simulink library "xsenslib"  (R2022a)
settings: Solver=VariableStepAuto  StartTime=0.0  StopTime=10.0  RelTol=1e-3
libraries: canmsglib x48, simulink x1
(part 1 of 2)
settings Model: Creator=rodri  LastModifiedBy=rodri

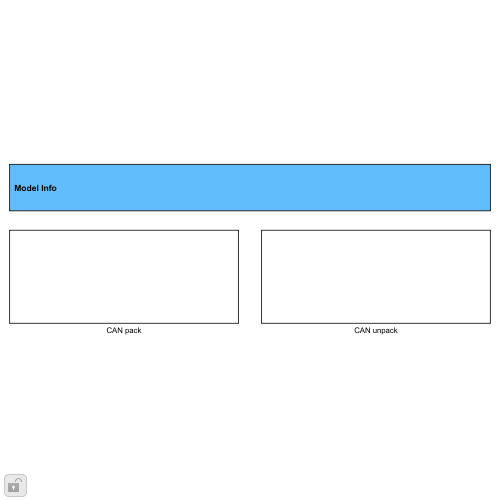
[thumbnail: Simulink's stored preview of the top-level diagram]
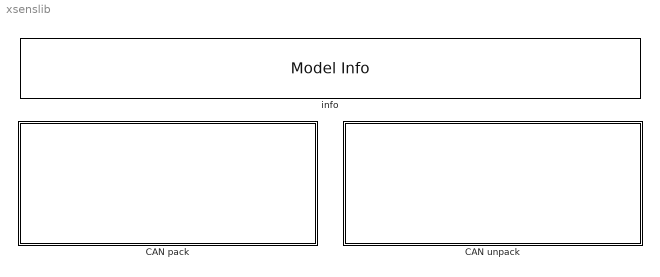
== system xsenslib ==
  CAN pack : Subsystem
  CAN unpack : Subsystem
  info : simulink/Model-Wide Utilities/Model Info  Frame=on  DisplayStringWithTags=SPEEDGOAT CAN Database Library for: xsens  HorizontalTextAlignment=Left  LeftAlignmentValue=0.01

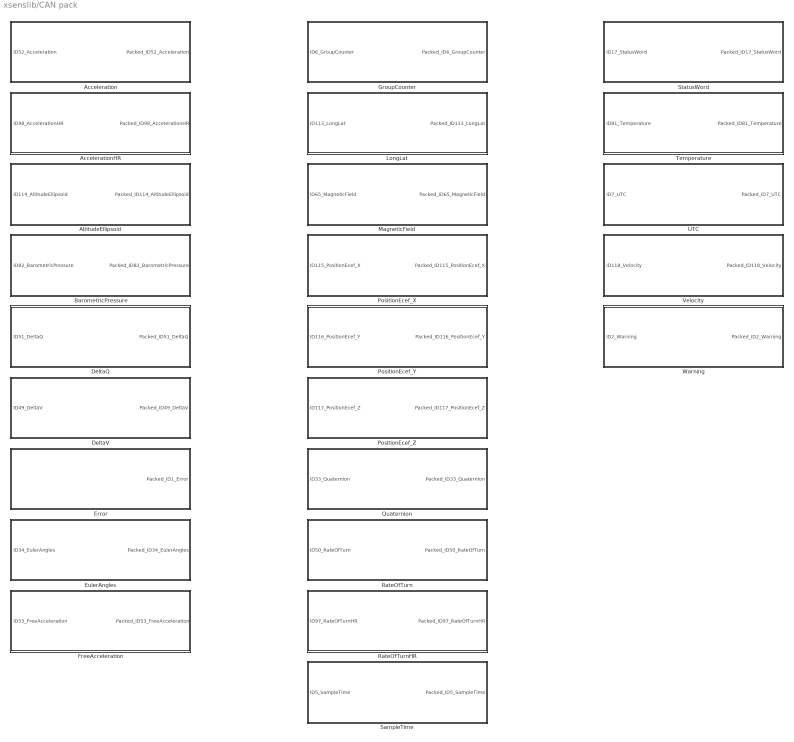
== system xsenslib/CAN pack ==
  Acceleration : Subsystem
  AccelerationHR : Subsystem
  AltitudeEllipsoid : Subsystem
  BarometricPressure : Subsystem
  DeltaQ : Subsystem
  DeltaV : Subsystem
  Error : Subsystem
  EulerAngles : Subsystem
  FreeAcceleration : Subsystem
  GroupCounter : Subsystem
  LongLat : Subsystem
  MagneticField : Subsystem
  PositionEcef_X : Subsystem
  PositionEcef_Y : Subsystem
  PositionEcef_Z : Subsystem
  Quaternion : Subsystem
  RateOfTurn : Subsystem
  RateOfTurnHR : Subsystem
  SampleTime : Subsystem
  StatusWord : Subsystem
  Temperature : Subsystem
  UTC : Subsystem
  Velocity : Subsystem
  Warning : Subsystem

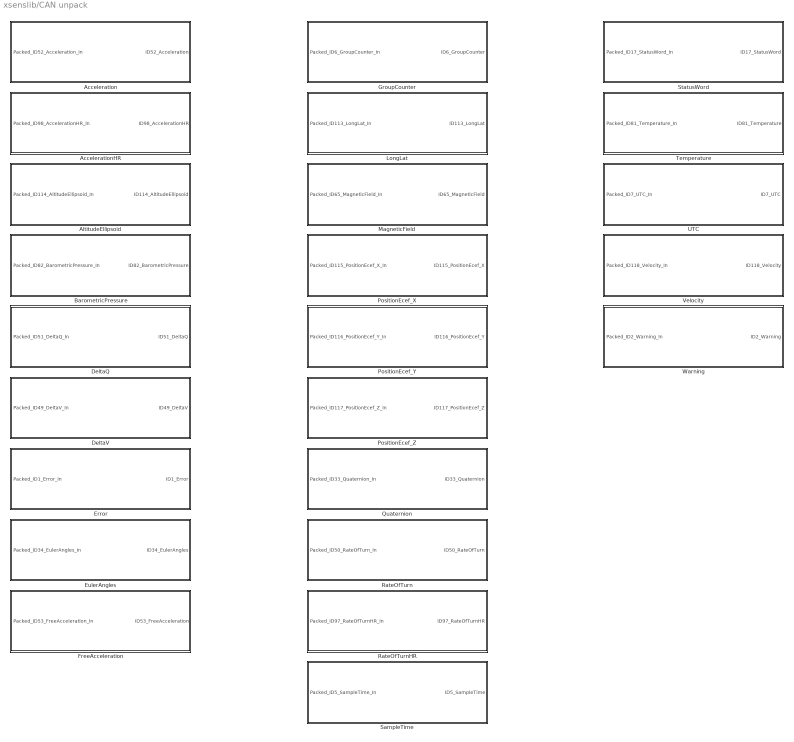
== system xsenslib/CAN unpack ==
  Acceleration : Subsystem
  AccelerationHR : Subsystem
  AltitudeEllipsoid : Subsystem
  BarometricPressure : Subsystem
  DeltaQ : Subsystem
  DeltaV : Subsystem
  Error : Subsystem
  EulerAngles : Subsystem
  FreeAcceleration : Subsystem
  GroupCounter : Subsystem
  LongLat : Subsystem
  MagneticField : Subsystem
  PositionEcef_X : Subsystem
  PositionEcef_Y : Subsystem
  PositionEcef_Z : Subsystem
  Quaternion : Subsystem
  RateOfTurn : Subsystem
  RateOfTurnHR : Subsystem
  SampleTime : Subsystem
  StatusWord : Subsystem
  Temperature : Subsystem
  UTC : Subsystem
  Velocity : Subsystem
  Warning : Subsystem

== system xsenslib/CAN pack/Acceleration ==
  In Bus Element : Inport  PortName=ID52_Acceleration  Element=accX
  In Bus Element1 : Inport  PortName=ID52_Acceleration  Element=accY
  In Bus Element2 : Inport  PortName=ID52_Acceleration  Element=accZ
  Acceleration : canmsglib/CAN Pack  CANdbFile=C:\Users\rodri\Dev\Projects\External\Tramontina\atlas\interface_models\xsens.dbc  MsgList=Acceleration  MsgName=Acceleration  MsgIDType=Standard (11-bit identifier)  MsgIdentifier=52  MsgLength=6  Remote=off  ApplyMinMax=off  BusOutput=on  SignalInfo={'accX','8','16','BE','signed','Standard','0','0.0039062','0','-100','100';'accY','24','16','BE','signed','Standard','0','0.0039062','0','-100','100';'accZ','40','16','BE','signed','Standard','0','0.0039062','0','-100','100'}
      settings: SourceProductBaseCode=XP,ME,VN  DataFormat=manually specified signals
  Packed_ID52_Acceleration : Outport
  wires:
  Acceleration/1 -> Packed_ID52_Acceleration/1
  In Bus Element/1 -> Acceleration/1
  In Bus Element1/1 -> Acceleration/2
  In Bus Element2/1 -> Acceleration/3

== system xsenslib/CAN pack/AccelerationHR ==
  In Bus Element : Inport  PortName=ID98_AccelerationHR  Element=HrAccX
  In Bus Element1 : Inport  PortName=ID98_AccelerationHR  Element=HrAccY
  In Bus Element2 : Inport  PortName=ID98_AccelerationHR  Element=HrAccZ
  AccelerationHR : canmsglib/CAN Pack  CANdbFile=C:\Users\rodri\Dev\Projects\External\Tramontina\atlas\interface_models\xsens.dbc  MsgList=AccelerationHR  MsgName=AccelerationHR  MsgIDType=Standard (11-bit identifier)  MsgIdentifier=98  MsgLength=6  Remote=off  ApplyMinMax=off  BusOutput=on  SignalInfo={'HrAccX','8','16','BE','signed','Standard','0','0.0039062','0','-100','100';'HrAccY','24','16','BE','signed','Standard','0','0.0039062','0','-100','100';'HrAccZ','40','16','BE','signed','Standard','0','0.0039062','0','-100','100'}
      settings: SourceProductBaseCode=XP,ME,VN  DataFormat=manually specified signals
  Packed_ID98_AccelerationHR : Outport
  wires:
  AccelerationHR/1 -> Packed_ID98_AccelerationHR/1
  In Bus Element/1 -> AccelerationHR/1
  In Bus Element1/1 -> AccelerationHR/2
  In Bus Element2/1 -> AccelerationHR/3

== system xsenslib/CAN pack/AltitudeEllipsoid ==
  In Bus Element : Inport  PortName=ID114_AltitudeEllipsoid  Element=altEllipsoid
  AltitudeEllipsoid : canmsglib/CAN Pack  CANdbFile=C:\Users\rodri\Dev\Projects\External\Tramontina\atlas\interface_models\xsens.dbc  MsgList=AltitudeEllipsoid  MsgName=AltitudeEllipsoid  MsgIDType=Standard (11-bit identifier)  MsgIdentifier=114  MsgLength=4  Remote=off  ApplyMinMax=off  BusOutput=on  SignalInfo={'altEllipsoid','24','32','BE','unsigned','Standard','0','3.0518e-05','0','0','50000'}
      settings: SourceProductBaseCode=XP,ME,VN  DataFormat=manually specified signals
  Packed_ID114_AltitudeEllipsoid : Outport
  wires:
  AltitudeEllipsoid/1 -> Packed_ID114_AltitudeEllipsoid/1
  In Bus Element/1 -> AltitudeEllipsoid/1

== system xsenslib/CAN pack/BarometricPressure ==
  In Bus Element : Inport  PortName=ID82_BarometricPressure  Element=Pressure
  BarometricPressure : canmsglib/CAN Pack  CANdbFile=C:\Users\rodri\Dev\Projects\External\Tramontina\atlas\interface_models\xsens.dbc  MsgList=BarometricPressure  MsgName=BarometricPressure  MsgIDType=Standard (11-bit identifier)  MsgIdentifier=82  MsgLength=4  Remote=off  ApplyMinMax=off  BusOutput=on  SignalInfo={'Pressure','24','32','BE','signed','Standard','0','3.0518e-05','0','30000','125000'}
      settings: SourceProductBaseCode=XP,ME,VN  DataFormat=manually specified signals
  Packed_ID82_BarometricPressure : Outport
  wires:
  BarometricPressure/1 -> Packed_ID82_BarometricPressure/1
  In Bus Element/1 -> BarometricPressure/1

== system xsenslib/CAN pack/DeltaQ ==
  In Bus Element : Inport  PortName=ID51_DeltaQ  Element=DeltaQ1
  In Bus Element1 : Inport  PortName=ID51_DeltaQ  Element=DeltaQ2
  In Bus Element2 : Inport  PortName=ID51_DeltaQ  Element=DeltaQ3
  In Bus Element3 : Inport  PortName=ID51_DeltaQ  Element=DeltaQ4
  DeltaQ : canmsglib/CAN Pack  CANdbFile=C:\Users\rodri\Dev\Projects\External\Tramontina\atlas\interface_models\xsens.dbc  MsgList=DeltaQ  MsgName=DeltaQ  MsgIDType=Standard (11-bit identifier)  MsgIdentifier=51  MsgLength=8  Remote=off  ApplyMinMax=off  BusOutput=on  SignalInfo={'DeltaQ1','8','16','BE','signed','Standard','0','3.0519e-05','0','-1','1';'DeltaQ2','24','16','BE','signed','Standard','0','3.0519e-05','0','-1','1';'DeltaQ3','40','16','BE','signed','Standard','0','3.0519e-05','0','-1','1';'DeltaQ4','56','16','BE','signed','Standard','0','3.0519e-05','0','-1','1'}
      settings: SourceProductBaseCode=XP,ME,VN  DataFormat=manually specified signals
  Packed_ID51_DeltaQ : Outport
  wires:
  DeltaQ/1 -> Packed_ID51_DeltaQ/1
  In Bus Element/1 -> DeltaQ/1
  In Bus Element1/1 -> DeltaQ/2
  In Bus Element2/1 -> DeltaQ/3
  In Bus Element3/1 -> DeltaQ/4

== system xsenslib/CAN pack/DeltaV ==
  In Bus Element : Inport  PortName=ID49_DeltaV  Element=Exponent
  In Bus Element1 : Inport  PortName=ID49_DeltaV  Element=X
  In Bus Element2 : Inport  PortName=ID49_DeltaV  Element=Y
  In Bus Element3 : Inport  PortName=ID49_DeltaV  Element=Z
  DeltaV : canmsglib/CAN Pack  CANdbFile=C:\Users\rodri\Dev\Projects\External\Tramontina\atlas\interface_models\xsens.dbc  MsgList=DeltaV  MsgName=DeltaV  MsgIDType=Standard (11-bit identifier)  MsgIdentifier=49  MsgLength=7  Remote=off  ApplyMinMax=off  BusOutput=on  SignalInfo={'Exponent','48','8','BE','unsigned','Standard','0','1','0','-Inf','Inf';'X','8','16','BE','signed','Standard','0','7.6294e-06','0','-0.25','0.25';'Y','24','16','BE','signed','Standard','0','7.6294e-06','0','-0.25','0.25';'Z','40','16','BE','signed','Standard','0','7.6294e-06','0','-0.25','0.25'}
      settings: SourceProductBaseCode=XP,ME,VN  DataFormat=manually specified signals
  Packed_ID49_DeltaV : Outport
  wires:
  DeltaV/1 -> Packed_ID49_DeltaV/1
  In Bus Element/1 -> DeltaV/1
  In Bus Element1/1 -> DeltaV/2
  In Bus Element2/1 -> DeltaV/3
  In Bus Element3/1 -> DeltaV/4

== system xsenslib/CAN pack/Error ==
  Error : canmsglib/CAN Pack  CANdbFile=C:\Users\rodri\Dev\Projects\External\Tramontina\atlas\interface_models\xsens.dbc  MsgList=Error  MsgName=Error  MsgIDType=Standard (11-bit identifier)  MsgIdentifier=1  MsgLength=1  Remote=off  ApplyMinMax=off  BusOutput=on  SignalInfo={}
      settings: SourceProductBaseCode=XP,ME,VN  DataFormat=manually specified signals
  Ground : Ground
  Packed_ID1_Error : Outport
  wires:
  Error/1 -> Packed_ID1_Error/1
  Ground/1 -> Error/1

== system xsenslib/CAN pack/EulerAngles ==
  In Bus Element : Inport  PortName=ID34_EulerAngles  Element=pitch
  In Bus Element1 : Inport  PortName=ID34_EulerAngles  Element=roll
  In Bus Element2 : Inport  PortName=ID34_EulerAngles  Element=yaw
  EulerAngles : canmsglib/CAN Pack  CANdbFile=C:\Users\rodri\Dev\Projects\External\Tramontina\atlas\interface_models\xsens.dbc  MsgList=EulerAngles  MsgName=EulerAngles  MsgIDType=Standard (11-bit identifier)  MsgIdentifier=34  MsgLength=6  Remote=off  ApplyMinMax=off  BusOutput=on  SignalInfo={'pitch','24','16','BE','signed','Standard','0','0.0078125','0','-90','90';'roll','8','16','BE','signed','Standard','0','0.0078125','0','-180','180';'yaw','40','16','BE','signed','Standard','0','0.0078125','0','-180','180'}
      settings: SourceProductBaseCode=XP,ME,VN  DataFormat=manually specified signals
  Packed_ID34_EulerAngles : Outport
  wires:
  EulerAngles/1 -> Packed_ID34_EulerAngles/1
  In Bus Element/1 -> EulerAngles/1
  In Bus Element1/1 -> EulerAngles/2
  In Bus Element2/1 -> EulerAngles/3

== system xsenslib/CAN pack/FreeAcceleration ==
  In Bus Element : Inport  PortName=ID53_FreeAcceleration  Element=FreeAccX
  In Bus Element1 : Inport  PortName=ID53_FreeAcceleration  Element=FreeAccY
  In Bus Element2 : Inport  PortName=ID53_FreeAcceleration  Element=FreeAccZ
  FreeAcceleration : canmsglib/CAN Pack  CANdbFile=C:\Users\rodri\Dev\Projects\External\Tramontina\atlas\interface_models\xsens.dbc  MsgList=FreeAcceleration  MsgName=FreeAcceleration  MsgIDType=Standard (11-bit identifier)  MsgIdentifier=53  MsgLength=6  Remote=off  ApplyMinMax=off  BusOutput=on  SignalInfo={'FreeAccX','8','16','BE','signed','Standard','0','0.0039062','0','-100','100';'FreeAccY','24','16','BE','signed','Standard','0','0.0039062','0','-100','100';'FreeAccZ','40','16','BE','signed','Standard','0','0.0039062','0','-100','100'}
      settings: SourceProductBaseCode=XP,ME,VN  DataFormat=manually specified signals
  Packed_ID53_FreeAcceleration : Outport
  wires:
  FreeAcceleration/1 -> Packed_ID53_FreeAcceleration/1
  In Bus Element/1 -> FreeAcceleration/1
  In Bus Element1/1 -> FreeAcceleration/2
  In Bus Element2/1 -> FreeAcceleration/3

== system xsenslib/CAN pack/GroupCounter ==
  In Bus Element : Inport  PortName=ID6_GroupCounter  Element=Counter
  GroupCounter : canmsglib/CAN Pack  CANdbFile=C:\Users\rodri\Dev\Projects\External\Tramontina\atlas\interface_models\xsens.dbc  MsgList=GroupCounter  MsgName=GroupCounter  MsgIDType=Standard (11-bit identifier)  MsgIdentifier=6  MsgLength=2  Remote=off  ApplyMinMax=off  BusOutput=on  SignalInfo={'Counter','8','16','BE','unsigned','Standard','0','1','0','-Inf','Inf'}
      settings: SourceProductBaseCode=XP,ME,VN  DataFormat=manually specified signals
  Packed_ID6_GroupCounter : Outport
  wires:
  GroupCounter/1 -> Packed_ID6_GroupCounter/1
  In Bus Element/1 -> GroupCounter/1

== system xsenslib/CAN pack/LongLat ==
  In Bus Element : Inport  PortName=ID113_LongLat  Element=latitude
  In Bus Element1 : Inport  PortName=ID113_LongLat  Element=longitude
  LongLat : canmsglib/CAN Pack  CANdbFile=C:\Users\rodri\Dev\Projects\External\Tramontina\atlas\interface_models\xsens.dbc  MsgList=LongLat  MsgName=LongLat  MsgIDType=Standard (11-bit identifier)  MsgIdentifier=113  MsgLength=8  Remote=off  ApplyMinMax=off  BusOutput=on  SignalInfo={'latitude','24','32','BE','signed','Standard','0','5.9605e-08','0','-90','90';'longitude','56','32','BE','signed','Standard','0','1.1921e-07','0','-180','180'}
      settings: SourceProductBaseCode=XP,ME,VN  DataFormat=manually specified signals
  Packed_ID113_LongLat : Outport
  wires:
  LongLat/1 -> Packed_ID113_LongLat/1
  In Bus Element/1 -> LongLat/1
  In Bus Element1/1 -> LongLat/2

== system xsenslib/CAN pack/MagneticField ==
  In Bus Element : Inport  PortName=ID65_MagneticField  Element=magX
  In Bus Element1 : Inport  PortName=ID65_MagneticField  Element=magY
  In Bus Element2 : Inport  PortName=ID65_MagneticField  Element=magZ
  MagneticField : canmsglib/CAN Pack  CANdbFile=C:\Users\rodri\Dev\Projects\External\Tramontina\atlas\interface_models\xsens.dbc  MsgList=MagneticField  MsgName=MagneticField  MsgIDType=Standard (11-bit identifier)  MsgIdentifier=65  MsgLength=6  Remote=off  ApplyMinMax=off  BusOutput=on  SignalInfo={'magX','8','16','BE','signed','Standard','0','0.00097656','0','-32','32';'magY','24','16','BE','signed','Standard','0','0.00097656','0','-32','32';'magZ','40','16','BE','signed','Standard','0','0.00097656','0','-32','32'}
      settings: SourceProductBaseCode=XP,ME,VN  DataFormat=manually specified signals
  Packed_ID65_MagneticField : Outport
  wires:
  MagneticField/1 -> Packed_ID65_MagneticField/1
  In Bus Element/1 -> MagneticField/1
  In Bus Element1/1 -> MagneticField/2
  In Bus Element2/1 -> MagneticField/3

== system xsenslib/CAN pack/PositionEcef_X ==
  In Bus Element : Inport  PortName=ID115_PositionEcef_X  Element=PositionEcef_X
  PositionEcef_X : canmsglib/CAN Pack  CANdbFile=C:\Users\rodri\Dev\Projects\External\Tramontina\atlas\interface_models\xsens.dbc  MsgList=PositionEcef_X  MsgName=PositionEcef_X  MsgIDType=Standard (11-bit identifier)  MsgIdentifier=115  MsgLength=4  Remote=off  ApplyMinMax=off  BusOutput=on  SignalInfo={'PositionEcef_X','24','32','BE','signed','Standard','0','0.0039062','0','-6500000','6500000'}
      settings: SourceProductBaseCode=XP,ME,VN  DataFormat=manually specified signals
  Packed_ID115_PositionEcef_X : Outport
  wires:
  PositionEcef_X/1 -> Packed_ID115_PositionEcef_X/1
  In Bus Element/1 -> PositionEcef_X/1

== system xsenslib/CAN pack/PositionEcef_Y ==
  In Bus Element : Inport  PortName=ID116_PositionEcef_Y  Element=PositionEcef_Y
  PositionEcef_Y : canmsglib/CAN Pack  CANdbFile=C:\Users\rodri\Dev\Projects\External\Tramontina\atlas\interface_models\xsens.dbc  MsgList=PositionEcef_Y  MsgName=PositionEcef_Y  MsgIDType=Standard (11-bit identifier)  MsgIdentifier=116  MsgLength=4  Remote=off  ApplyMinMax=off  BusOutput=on  SignalInfo={'PositionEcef_Y','24','32','BE','signed','Standard','0','0.0039062','0','-6500000','6500000'}
      settings: SourceProductBaseCode=XP,ME,VN  DataFormat=manually specified signals
  Packed_ID116_PositionEcef_Y : Outport
  wires:
  PositionEcef_Y/1 -> Packed_ID116_PositionEcef_Y/1
  In Bus Element/1 -> PositionEcef_Y/1

== system xsenslib/CAN pack/PositionEcef_Z ==
  In Bus Element : Inport  PortName=ID117_PositionEcef_Z  Element=PositionEcef_Z
  PositionEcef_Z : canmsglib/CAN Pack  CANdbFile=C:\Users\rodri\Dev\Projects\External\Tramontina\atlas\interface_models\xsens.dbc  MsgList=PositionEcef_Z  MsgName=PositionEcef_Z  MsgIDType=Standard (11-bit identifier)  MsgIdentifier=117  MsgLength=4  Remote=off  ApplyMinMax=off  BusOutput=on  SignalInfo={'PositionEcef_Z','24','32','BE','signed','Standard','0','0.0039062','0','-6500000','6500000'}
      settings: SourceProductBaseCode=XP,ME,VN  DataFormat=manually specified signals
  Packed_ID117_PositionEcef_Z : Outport
  wires:
  PositionEcef_Z/1 -> Packed_ID117_PositionEcef_Z/1
  In Bus Element/1 -> PositionEcef_Z/1

== system xsenslib/CAN pack/Quaternion ==
  In Bus Element : Inport  PortName=ID33_Quaternion  Element=Q1
  In Bus Element1 : Inport  PortName=ID33_Quaternion  Element=Q2
  In Bus Element2 : Inport  PortName=ID33_Quaternion  Element=Q3
  In Bus Element3 : Inport  PortName=ID33_Quaternion  Element=Q4
  Quaternion : canmsglib/CAN Pack  CANdbFile=C:\Users\rodri\Dev\Projects\External\Tramontina\atlas\interface_models\xsens.dbc  MsgList=Quaternion  MsgName=Quaternion  MsgIDType=Standard (11-bit identifier)  MsgIdentifier=33  MsgLength=8  Remote=off  ApplyMinMax=off  BusOutput=on  SignalInfo={'Q1','8','16','BE','signed','Standard','0','3.0518e-05','0','-1','1';'Q2','24','16','BE','signed','Standard','0','3.0518e-05','0','-1','1';'Q3','40','16','BE','signed','Standard','0','3.0518e-05','0','-1','1';'Q4','56','16','BE','signed','Standard','0','3.0518e-05','0','-Inf','Inf'}
      settings: SourceProductBaseCode=XP,ME,VN  DataFormat=manually specified signals
  Packed_ID33_Quaternion : Outport
  wires:
  Quaternion/1 -> Packed_ID33_Quaternion/1
  In Bus Element/1 -> Quaternion/1
  In Bus Element1/1 -> Quaternion/2
  In Bus Element2/1 -> Quaternion/3
  In Bus Element3/1 -> Quaternion/4

== system xsenslib/CAN pack/RateOfTurn ==
  In Bus Element : Inport  PortName=ID50_RateOfTurn  Element=gyrX
  In Bus Element1 : Inport  PortName=ID50_RateOfTurn  Element=gyrY
  In Bus Element2 : Inport  PortName=ID50_RateOfTurn  Element=gyrZ
  RateOfTurn : canmsglib/CAN Pack  CANdbFile=C:\Users\rodri\Dev\Projects\External\Tramontina\atlas\interface_models\xsens.dbc  MsgList=RateOfTurn  MsgName=RateOfTurn  MsgIDType=Standard (11-bit identifier)  MsgIdentifier=50  MsgLength=6  Remote=off  ApplyMinMax=off  BusOutput=on  SignalInfo={'gyrX','8','16','BE','signed','Standard','0','0.0019531','0','-Inf','Inf';'gyrY','24','16','BE','signed','Standard','0','0.0019531','0','-Inf','Inf';'gyrZ','40','16','BE','signed','Standard','0','0.0019531','0','-Inf','Inf'}
      settings: SourceProductBaseCode=XP,ME,VN  DataFormat=manually specified signals
  Packed_ID50_RateOfTurn : Outport
  wires:
  RateOfTurn/1 -> Packed_ID50_RateOfTurn/1
  In Bus Element/1 -> RateOfTurn/1
  In Bus Element1/1 -> RateOfTurn/2
  In Bus Element2/1 -> RateOfTurn/3

== system xsenslib/CAN pack/RateOfTurnHR ==
  In Bus Element : Inport  PortName=ID97_RateOfTurnHR  Element=HrGyrX
  In Bus Element1 : Inport  PortName=ID97_RateOfTurnHR  Element=HrGyrY
  In Bus Element2 : Inport  PortName=ID97_RateOfTurnHR  Element=HrGyrZ
  RateOfTurnHR : canmsglib/CAN Pack  CANdbFile=C:\Users\rodri\Dev\Projects\External\Tramontina\atlas\interface_models\xsens.dbc  MsgList=RateOfTurnHR  MsgName=RateOfTurnHR  MsgIDType=Standard (11-bit identifier)  MsgIdentifier=97  MsgLength=6  Remote=off  ApplyMinMax=off  BusOutput=on  SignalInfo={'HrGyrX','8','16','BE','signed','Standard','0','0.0019531','0','-Inf','Inf';'HrGyrY','24','16','BE','signed','Standard','0','0.0019531','0','-Inf','Inf';'HrGyrZ','40','16','BE','signed','Standard','0','0.0019531','0','-Inf','Inf'}
      settings: SourceProductBaseCode=XP,ME,VN  DataFormat=manually specified signals
  Packed_ID97_RateOfTurnHR : Outport
  wires:
  RateOfTurnHR/1 -> Packed_ID97_RateOfTurnHR/1
  In Bus Element/1 -> RateOfTurnHR/1
  In Bus Element1/1 -> RateOfTurnHR/2
  In Bus Element2/1 -> RateOfTurnHR/3

== system xsenslib/CAN pack/SampleTime ==
  In Bus Element : Inport  PortName=ID5_SampleTime  Element=Timestamp
  SampleTime : canmsglib/CAN Pack  CANdbFile=C:\Users\rodri\Dev\Projects\External\Tramontina\atlas\interface_models\xsens.dbc  MsgList=SampleTime  MsgName=SampleTime  MsgIDType=Standard (11-bit identifier)  MsgIdentifier=5  MsgLength=4  Remote=off  ApplyMinMax=off  BusOutput=on  SignalInfo={'Timestamp','24','32','BE','unsigned','Standard','0','1','0','-Inf','Inf'}
      settings: SourceProductBaseCode=XP,ME,VN  DataFormat=manually specified signals
  Packed_ID5_SampleTime : Outport
  wires:
  SampleTime/1 -> Packed_ID5_SampleTime/1
  In Bus Element/1 -> SampleTime/1

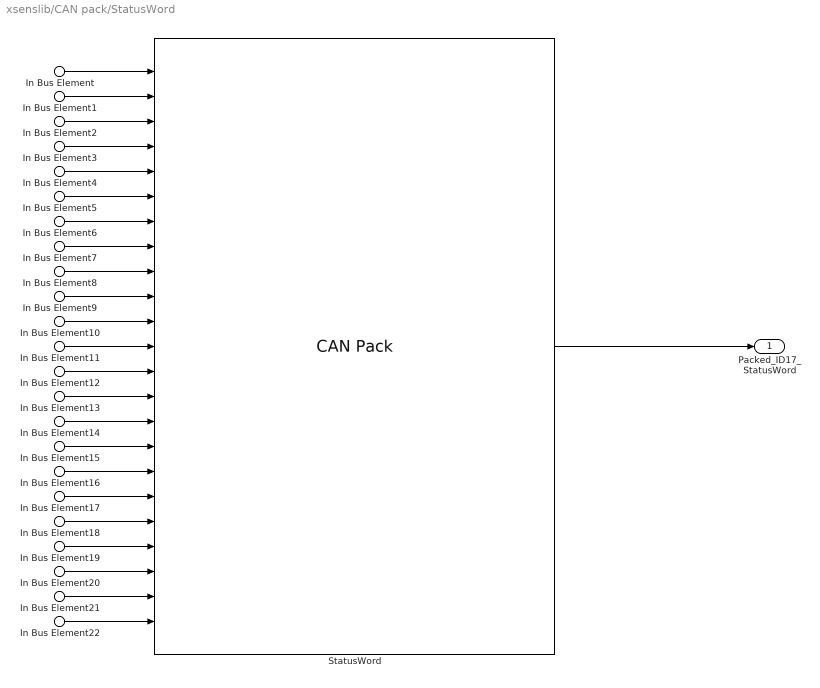
== system xsenslib/CAN pack/StatusWord ==
  In Bus Element : Inport  PortName=ID17_StatusWord  Element=ClipAccX
  In Bus Element1 : Inport  PortName=ID17_StatusWord  Element=ClipAccY
  In Bus Element2 : Inport  PortName=ID17_StatusWord  Element=ClipAccZ
  In Bus Element3 : Inport  PortName=ID17_StatusWord  Element=ClipGyrX
  In Bus Element4 : Inport  PortName=ID17_StatusWord  Element=ClipGyrY
  In Bus Element5 : Inport  PortName=ID17_StatusWord  Element=ClipGyrZ
  In Bus Element6 : Inport  PortName=ID17_StatusWord  Element=ClipMagX
  In Bus Element7 : Inport  PortName=ID17_StatusWord  Element=ClipMagY
  In Bus Element8 : Inport  PortName=ID17_StatusWord  Element=ClipMagZ
  In Bus Element9 : Inport  PortName=ID17_StatusWord  Element=ClippingDetected
  In Bus Element10 : Inport  PortName=ID17_StatusWord  Element=ExternalClockSynced
  In Bus Element11 : Inport  PortName=ID17_StatusWord  Element=FilterMode
  In Bus Element12 : Inport  PortName=ID17_StatusWord  Element=GpsValid
  In Bus Element13 : Inport  PortName=ID17_StatusWord  Element=HaveGnssTimePulse
  In Bus Element14 : Inport  PortName=ID17_StatusWord  Element=Interpolated
  In Bus Element15 : Inport  PortName=ID17_StatusWord  Element=NoRotation
  In Bus Element16 : Inport  PortName=ID17_StatusWord  Element=OrientationValid
  In Bus Element17 : Inport  PortName=ID17_StatusWord  Element=RepresentativeMotion
  In Bus Element18 : Inport  PortName=ID17_StatusWord  Element=Retransmitted
  In Bus Element19 : Inport  PortName=ID17_StatusWord  Element=RtkStatus
  In Bus Element20 : Inport  PortName=ID17_StatusWord  Element=SelfTestOk
  In Bus Element21 : Inport  PortName=ID17_StatusWord  Element=SyncIn
  In Bus Element22 : Inport  PortName=ID17_StatusWord  Element=SyncOut
  StatusWord : canmsglib/CAN Pack  CANdbFile=C:\Users\rodri\Dev\Projects\External\Tramontina\atlas\interface_models\xsens.dbc  MsgList=StatusWord  MsgName=StatusWord  MsgIDType=Standard (11-bit identifier)  MsgIdentifier=17  MsgLength=4  Remote=off  ApplyMinMax=off  BusOutput=on  SignalInfo={'ClipAccX','16','1','LE','unsigned','Standard','0','1','0','0','1';'ClipAccY','17','1','LE','unsigned','Standard','0','1','0','0','1';'ClipAccZ','18','1','LE','unsigned','Standard','0','1','0','0','1';'ClipGyrX','19','1','LE','unsigned','Standard','0','1','0','0','1';'ClipGyrY','20','1','LE','unsigned','Standard','0','1','0','0','1';'ClipGyrZ','21','1','LE','unsigned','Standard','0','1','0','0','1';'ClipMagX','22','1','LE','unsigned','Standard','0','1','0','0','1';'ClipMagY','23','1','LE','unsigned','Standard','0','1','0','0','1';'ClipMagZ','8','1','LE','unsigned','Standard','0','1','0','0','1';'ClippingDetected','11','1','LE','unsigned','Standard','0','1','0','0','1';'ExternalClockSynced','30','1','LE','unsigned','Standard','0','1','0','0','1';'FilterMode','15','3','BE','unsigned','Standard','0','1','0','0','1';'GpsValid','26','1','LE','unsigned','Standard','0','1','0','0','1';'HaveGnssTimePulse','2','1','LE','unsigned','Standard','0','1','0','0','1';'Interpolated','12','1','LE','unsigned','Standard','0','1','0','0','1';'NoRotation','27','2','BE','unsigned','Standard','0','1','0','0','3';'OrientationValid','25','1','LE','unsigned','Standard','0','1','0','0','1';'RepresentativeMotion','29','1','LE','unsigned','Standard','0','1','0','0','1';'Retransmitted','10','1','LE','unsigned','Standard','0','1','0','0','1';'RtkStatus','3','2','BE','unsigned','Standard','0','1','0','0','1';'SelfTestOk','24','1','LE','unsigned','Standard','0','1','0','0','1';'SyncIn','13','1','LE','unsigned','Standard','0','1','0','0','1';'SyncOut','14','1','LE','unsigned','Standard','0','1','0','0','1'}
      settings: SourceProductBaseCode=XP,ME,VN  DataFormat=manually specified signals
  Packed_ID17_StatusWord : Outport
  wires:
  StatusWord/1 -> Packed_ID17_StatusWord/1
  In Bus Element/1 -> StatusWord/1
  In Bus Element1/1 -> StatusWord/2
  In Bus Element2/1 -> StatusWord/3
  In Bus Element3/1 -> StatusWord/4
  In Bus Element4/1 -> StatusWord/5
  In Bus Element5/1 -> StatusWord/6
  In Bus Element6/1 -> StatusWord/7
  In Bus Element7/1 -> StatusWord/8
  In Bus Element8/1 -> StatusWord/9
  In Bus Element9/1 -> StatusWord/10
  In Bus Element10/1 -> StatusWord/11
  In Bus Element11/1 -> StatusWord/12
  In Bus Element12/1 -> StatusWord/13
  In Bus Element13/1 -> StatusWord/14
  In Bus Element14/1 -> StatusWord/15
  In Bus Element15/1 -> StatusWord/16
  In Bus Element16/1 -> StatusWord/17
  In Bus Element17/1 -> StatusWord/18
  In Bus Element18/1 -> StatusWord/19
  In Bus Element19/1 -> StatusWord/20
  In Bus Element20/1 -> StatusWord/21
  In Bus Element21/1 -> StatusWord/22
  In Bus Element22/1 -> StatusWord/23

== system xsenslib/CAN pack/Temperature ==
  In Bus Element : Inport  PortName=ID81_Temperature  Element=Temperature
  Temperature : canmsglib/CAN Pack  CANdbFile=C:\Users\rodri\Dev\Projects\External\Tramontina\atlas\interface_models\xsens.dbc  MsgList=Temperature  MsgName=Temperature  MsgIDType=Standard (11-bit identifier)  MsgIdentifier=81  MsgLength=2  Remote=off  ApplyMinMax=off  BusOutput=on  SignalInfo={'Temperature','8','16','BE','signed','Standard','0','0.0039062','0','-40','85'}
      settings: SourceProductBaseCode=XP,ME,VN  DataFormat=manually specified signals
  Packed_ID81_Temperature : Outport
  wires:
  Temperature/1 -> Packed_ID81_Temperature/1
  In Bus Element/1 -> Temperature/1

== system xsenslib/CAN pack/UTC ==
  In Bus Element : Inport  PortName=ID7_UTC  Element=day
  In Bus Element1 : Inport  PortName=ID7_UTC  Element=hour
  In Bus Element2 : Inport  PortName=ID7_UTC  Element=minute
  In Bus Element3 : Inport  PortName=ID7_UTC  Element=month
  In Bus Element4 : Inport  PortName=ID7_UTC  Element=second
  In Bus Element5 : Inport  PortName=ID7_UTC  Element=tenthms
  In Bus Element6 : Inport  PortName=ID7_UTC  Element=year
  UTC : canmsglib/CAN Pack  CANdbFile=C:\Users\rodri\Dev\Projects\External\Tramontina\atlas\interface_models\xsens.dbc  MsgList=UTC  MsgName=UTC  MsgIDType=Standard (11-bit identifier)  MsgIdentifier=7  MsgLength=8  Remote=off  ApplyMinMax=off  BusOutput=on  SignalInfo={'day','16','8','BE','unsigned','Standard','0','1','0','1','31';'hour','24','8','BE','unsigned','Standard','0','1','0','0','24';'minute','32','8','BE','unsigned','Standard','0','1','0','0','60';'month','8','8','BE','unsigned','Standard','0','1','0','1','12';'second','40','8','BE','unsigned','Standard','0','1','0','0','60';'tenthms','56','16','BE','unsigned','Standard','0','1','0','-Inf','Inf';'year','0','8','BE','unsigned','Standard','0','1','0','-Inf','Inf'}
      settings: SourceProductBaseCode=XP,ME,VN  DataFormat=manually specified signals
  Packed_ID7_UTC : Outport
  wires:
  UTC/1 -> Packed_ID7_UTC/1
  In Bus Element/1 -> UTC/1
  In Bus Element1/1 -> UTC/2
  In Bus Element2/1 -> UTC/3
  In Bus Element3/1 -> UTC/4
  In Bus Element4/1 -> UTC/5
  In Bus Element5/1 -> UTC/6
  In Bus Element6/1 -> UTC/7

== system xsenslib/CAN pack/Velocity ==
  In Bus Element : Inport  PortName=ID118_Velocity  Element=velX
  In Bus Element1 : Inport  PortName=ID118_Velocity  Element=velY
  In Bus Element2 : Inport  PortName=ID118_Velocity  Element=velZ
  Velocity : canmsglib/CAN Pack  CANdbFile=C:\Users\rodri\Dev\Projects\External\Tramontina\atlas\interface_models\xsens.dbc  MsgList=Velocity  MsgName=Velocity  MsgIDType=Standard (11-bit identifier)  MsgIdentifier=118  MsgLength=6  Remote=off  ApplyMinMax=off  BusOutput=on  SignalInfo={'velX','8','16','BE','signed','Standard','0','0.015625','0','-500','500';'velY','24','16','BE','signed','Standard','0','0.015625','0','-500','500';'velZ','40','16','BE','signed','Standard','0','0.015625','0','-500','500'}
      settings: SourceProductBaseCode=XP,ME,VN  DataFormat=manually specified signals
  Packed_ID118_Velocity : Outport
  wires:
  Velocity/1 -> Packed_ID118_Velocity/1
  In Bus Element/1 -> Velocity/1
  In Bus Element1/1 -> Velocity/2
  In Bus Element2/1 -> Velocity/3

== system xsenslib/CAN pack/Warning ==
  In Bus Element : Inport  PortName=ID2_Warning  Element=WarningCode
  Warning : canmsglib/CAN Pack  CANdbFile=C:\Users\rodri\Dev\Projects\External\Tramontina\atlas\interface_models\xsens.dbc  MsgList=Warning  MsgName=Warning  MsgIDType=Standard (11-bit identifier)  MsgIdentifier=2  MsgLength=1  Remote=off  ApplyMinMax=off  BusOutput=on  SignalInfo={'WarningCode','0','8','BE','unsigned','Standard','0','1','0','-Inf','Inf'}
      settings: SourceProductBaseCode=XP,ME,VN  DataFormat=manually specified signals
  Packed_ID2_Warning : Outport
  wires:
  Warning/1 -> Packed_ID2_Warning/1
  In Bus Element/1 -> Warning/1

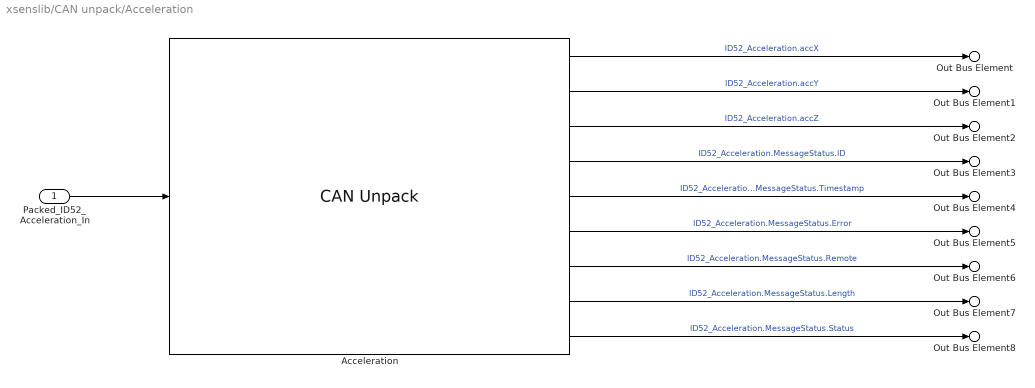
== system xsenslib/CAN unpack/Acceleration ==
  Packed_ID52_Acceleration_In : Inport
  Acceleration : canmsglib/CAN Unpack  CANdbFile=C:\Users\rodri\Dev\Projects\External\Tramontina\atlas\interface_models\xsens.dbc  MsgList=Acceleration  MsgName=Acceleration  MsgIDType=Standard (11-bit identifier)  MsgIdentifier=52  MsgLength=6  SignalInfo={'accX','8','16','BE','signed','Standard','0','0.0039062','0','-100','100';'accY','24','16','BE','signed','Standard','0','0.0039062','0','-100','100';'accZ','40','16','BE','signed','Standard','0','0.0039062','0','-100','100'}  IDPort=on  TimestampPort=on  ErrorPort=on  RemotePort=on  LengthPort=on  StatusPort=on  ApplyMinMax=off
      settings: SourceProductBaseCode=XP,ME,VN
  Out Bus Element : Outport  PortName=ID52_Acceleration  Element=accX
  Out Bus Element1 : Outport  PortName=ID52_Acceleration  Element=accY
  Out Bus Element2 : Outport  PortName=ID52_Acceleration  Element=accZ
  Out Bus Element3 : Outport  PortName=ID52_Acceleration  Element=MessageStatus.ID
  Out Bus Element4 : Outport  PortName=ID52_Acceleration  Element=MessageStatus.Timestamp
  Out Bus Element5 : Outport  PortName=ID52_Acceleration  Element=MessageStatus.Error
  Out Bus Element6 : Outport  PortName=ID52_Acceleration  Element=MessageStatus.Remote
  Out Bus Element7 : Outport  PortName=ID52_Acceleration  Element=MessageStatus.Length
  Out Bus Element8 : Outport  PortName=ID52_Acceleration  Element=MessageStatus.Status
  wires:
  Packed_ID52_Acceleration_In/1 -> Acceleration/1
  Acceleration/1 -> Out Bus Element/1  "ID52_Acceleration.accX"
  Acceleration/2 -> Out Bus Element1/1  "ID52_Acceleration.accY"
  Acceleration/3 -> Out Bus Element2/1  "ID52_Acceleration.accZ"
  Acceleration/4 -> Out Bus Element3/1  "ID52_Acceleration.MessageStatus.ID"
  Acceleration/5 -> Out Bus Element4/1  "ID52_Acceleration.MessageStatus.Timestamp"
  Acceleration/6 -> Out Bus Element5/1  "ID52_Acceleration.MessageStatus.Error"
  Acceleration/7 -> Out Bus Element6/1  "ID52_Acceleration.MessageStatus.Remote"
  Acceleration/8 -> Out Bus Element7/1  "ID52_Acceleration.MessageStatus.Length"
  Acceleration/9 -> Out Bus Element8/1  "ID52_Acceleration.MessageStatus.Status"

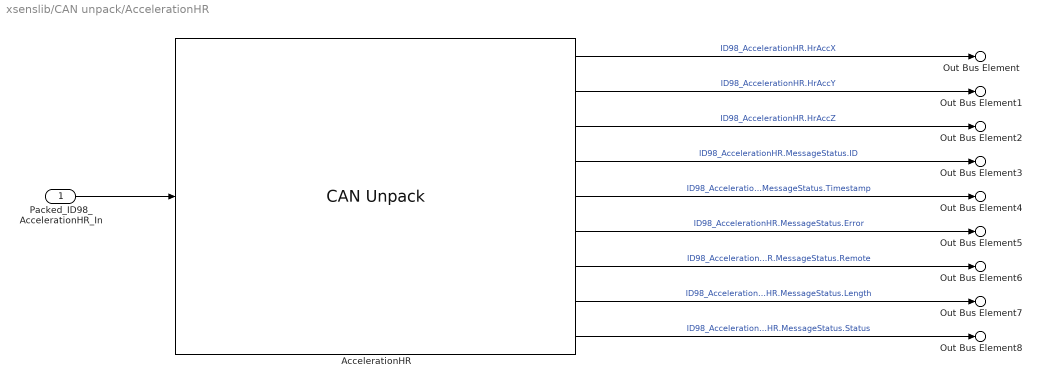
== system xsenslib/CAN unpack/AccelerationHR ==
  Packed_ID98_AccelerationHR_In : Inport
  AccelerationHR : canmsglib/CAN Unpack  CANdbFile=C:\Users\rodri\Dev\Projects\External\Tramontina\atlas\interface_models\xsens.dbc  MsgList=AccelerationHR  MsgName=AccelerationHR  MsgIDType=Standard (11-bit identifier)  MsgIdentifier=98  MsgLength=6  SignalInfo={'HrAccX','8','16','BE','signed','Standard','0','0.0039062','0','-100','100';'HrAccY','24','16','BE','signed','Standard','0','0.0039062','0','-100','100';'HrAccZ','40','16','BE','signed','Standard','0','0.0039062','0','-100','100'}  IDPort=on  TimestampPort=on  ErrorPort=on  RemotePort=on  LengthPort=on  StatusPort=on  ApplyMinMax=off
      settings: SourceProductBaseCode=XP,ME,VN
  Out Bus Element : Outport  PortName=ID98_AccelerationHR  Element=HrAccX
  Out Bus Element1 : Outport  PortName=ID98_AccelerationHR  Element=HrAccY
  Out Bus Element2 : Outport  PortName=ID98_AccelerationHR  Element=HrAccZ
  Out Bus Element3 : Outport  PortName=ID98_AccelerationHR  Element=MessageStatus.ID
  Out Bus Element4 : Outport  PortName=ID98_AccelerationHR  Element=MessageStatus.Timestamp
  Out Bus Element5 : Outport  PortName=ID98_AccelerationHR  Element=MessageStatus.Error
  Out Bus Element6 : Outport  PortName=ID98_AccelerationHR  Element=MessageStatus.Remote
  Out Bus Element7 : Outport  PortName=ID98_AccelerationHR  Element=MessageStatus.Length
  Out Bus Element8 : Outport  PortName=ID98_AccelerationHR  Element=MessageStatus.Status
  wires:
  Packed_ID98_AccelerationHR_In/1 -> AccelerationHR/1
  AccelerationHR/1 -> Out Bus Element/1  "ID98_AccelerationHR.HrAccX"
  AccelerationHR/2 -> Out Bus Element1/1  "ID98_AccelerationHR.HrAccY"
  AccelerationHR/3 -> Out Bus Element2/1  "ID98_AccelerationHR.HrAccZ"
  AccelerationHR/4 -> Out Bus Element3/1  "ID98_AccelerationHR.MessageStatus.ID"
  AccelerationHR/5 -> Out Bus Element4/1  "ID98_AccelerationHR.MessageStatus.Timestamp"
  AccelerationHR/6 -> Out Bus Element5/1  "ID98_AccelerationHR.MessageStatus.Error"
  AccelerationHR/7 -> Out Bus Element6/1  "ID98_AccelerationHR.MessageStatus.Remote"
  AccelerationHR/8 -> Out Bus Element7/1  "ID98_AccelerationHR.MessageStatus.Length"
  AccelerationHR/9 -> Out Bus Element8/1  "ID98_AccelerationHR.MessageStatus.Status"

== system xsenslib/CAN unpack/AltitudeEllipsoid ==
  Packed_ID114_AltitudeEllipsoid_In : Inport
  AltitudeEllipsoid : canmsglib/CAN Unpack  CANdbFile=C:\Users\rodri\Dev\Projects\External\Tramontina\atlas\interface_models\xsens.dbc  MsgList=AltitudeEllipsoid  MsgName=AltitudeEllipsoid  MsgIDType=Standard (11-bit identifier)  MsgIdentifier=114  MsgLength=4  SignalInfo={'altEllipsoid','24','32','BE','unsigned','Standard','0','3.0518e-05','0','0','50000'}  IDPort=on  TimestampPort=on  ErrorPort=on  RemotePort=on  LengthPort=on  StatusPort=on  ApplyMinMax=off
      settings: SourceProductBaseCode=XP,ME,VN
  Out Bus Element : Outport  PortName=ID114_AltitudeEllipsoid  Element=altEllipsoid
  Out Bus Element1 : Outport  PortName=ID114_AltitudeEllipsoid  Element=MessageStatus.ID
  Out Bus Element2 : Outport  PortName=ID114_AltitudeEllipsoid  Element=MessageStatus.Timestamp
  Out Bus Element3 : Outport  PortName=ID114_AltitudeEllipsoid  Element=MessageStatus.Error
  Out Bus Element4 : Outport  PortName=ID114_AltitudeEllipsoid  Element=MessageStatus.Remote
  Out Bus Element5 : Outport  PortName=ID114_AltitudeEllipsoid  Element=MessageStatus.Length
  Out Bus Element6 : Outport  PortName=ID114_AltitudeEllipsoid  Element=MessageStatus.Status
  wires:
  Packed_ID114_AltitudeEllipsoid_In/1 -> AltitudeEllipsoid/1
  AltitudeEllipsoid/1 -> Out Bus Element/1  "ID114_AltitudeEllipsoid.altEllipsoid"
  AltitudeEllipsoid/2 -> Out Bus Element1/1  "ID114_AltitudeEllipsoid.MessageStatus.ID"
  AltitudeEllipsoid/3 -> Out Bus Element2/1  "ID114_AltitudeEllipsoid.MessageStatus.Timestamp"
  AltitudeEllipsoid/4 -> Out Bus Element3/1  "ID114_AltitudeEllipsoid.MessageStatus.Error"
  AltitudeEllipsoid/5 -> Out Bus Element4/1  "ID114_AltitudeEllipsoid.MessageStatus.Remote"
  AltitudeEllipsoid/6 -> Out Bus Element5/1  "ID114_AltitudeEllipsoid.MessageStatus.Length"
  AltitudeEllipsoid/7 -> Out Bus Element6/1  "ID114_AltitudeEllipsoid.MessageStatus.Status"

== system xsenslib/CAN unpack/BarometricPressure ==
  Packed_ID82_BarometricPressure_In : Inport
  BarometricPressure : canmsglib/CAN Unpack  CANdbFile=C:\Users\rodri\Dev\Projects\External\Tramontina\atlas\interface_models\xsens.dbc  MsgList=BarometricPressure  MsgName=BarometricPressure  MsgIDType=Standard (11-bit identifier)  MsgIdentifier=82  MsgLength=4  SignalInfo={'Pressure','24','32','BE','signed','Standard','0','3.0518e-05','0','30000','125000'}  IDPort=on  TimestampPort=on  ErrorPort=on  RemotePort=on  LengthPort=on  StatusPort=on  ApplyMinMax=off
      settings: SourceProductBaseCode=XP,ME,VN
  Out Bus Element : Outport  PortName=ID82_BarometricPressure  Element=Pressure
  Out Bus Element1 : Outport  PortName=ID82_BarometricPressure  Element=MessageStatus.ID
  Out Bus Element2 : Outport  PortName=ID82_BarometricPressure  Element=MessageStatus.Timestamp
  Out Bus Element3 : Outport  PortName=ID82_BarometricPressure  Element=MessageStatus.Error
  Out Bus Element4 : Outport  PortName=ID82_BarometricPressure  Element=MessageStatus.Remote
  Out Bus Element5 : Outport  PortName=ID82_BarometricPressure  Element=MessageStatus.Length
  Out Bus Element6 : Outport  PortName=ID82_BarometricPressure  Element=MessageStatus.Status
  wires:
  Packed_ID82_BarometricPressure_In/1 -> BarometricPressure/1
  BarometricPressure/1 -> Out Bus Element/1  "ID82_BarometricPressure.Pressure"
  BarometricPressure/2 -> Out Bus Element1/1  "ID82_BarometricPressure.MessageStatus.ID"
  BarometricPressure/3 -> Out Bus Element2/1  "ID82_BarometricPressure.MessageStatus.Timestamp"
  BarometricPressure/4 -> Out Bus Element3/1  "ID82_BarometricPressure.MessageStatus.Error"
  BarometricPressure/5 -> Out Bus Element4/1  "ID82_BarometricPressure.MessageStatus.Remote"
  BarometricPressure/6 -> Out Bus Element5/1  "ID82_BarometricPressure.MessageStatus.Length"
  BarometricPressure/7 -> Out Bus Element6/1  "ID82_BarometricPressure.MessageStatus.Status"

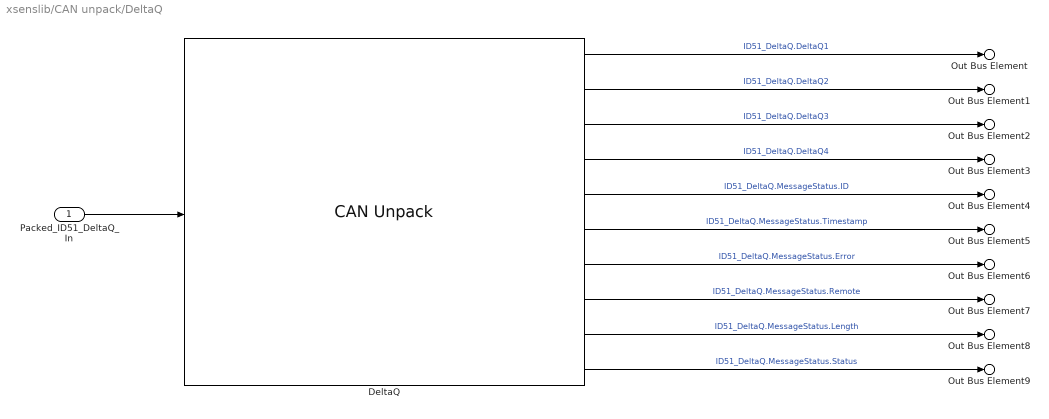
== system xsenslib/CAN unpack/DeltaQ ==
  Packed_ID51_DeltaQ_In : Inport
  DeltaQ : canmsglib/CAN Unpack  CANdbFile=C:\Users\rodri\Dev\Projects\External\Tramontina\atlas\interface_models\xsens.dbc  MsgList=DeltaQ  MsgName=DeltaQ  MsgIDType=Standard (11-bit identifier)  MsgIdentifier=51  MsgLength=8  SignalInfo={'DeltaQ1','8','16','BE','signed','Standard','0','3.0519e-05','0','-1','1';'DeltaQ2','24','16','BE','signed','Standard','0','3.0519e-05','0','-1','1';'DeltaQ3','40','16','BE','signed','Standard','0','3.0519e-05','0','-1','1';'DeltaQ4','56','16','BE','signed','Standard','0','3.0519e-05','0','-1','1'}  IDPort=on  TimestampPort=on  ErrorPort=on  RemotePort=on  LengthPort=on  StatusPort=on  ApplyMinMax=off
      settings: SourceProductBaseCode=XP,ME,VN
  Out Bus Element : Outport  PortName=ID51_DeltaQ  Element=DeltaQ1
  Out Bus Element1 : Outport  PortName=ID51_DeltaQ  Element=DeltaQ2
  Out Bus Element2 : Outport  PortName=ID51_DeltaQ  Element=DeltaQ3
  Out Bus Element3 : Outport  PortName=ID51_DeltaQ  Element=DeltaQ4
  Out Bus Element4 : Outport  PortName=ID51_DeltaQ  Element=MessageStatus.ID
  Out Bus Element5 : Outport  PortName=ID51_DeltaQ  Element=MessageStatus.Timestamp
  Out Bus Element6 : Outport  PortName=ID51_DeltaQ  Element=MessageStatus.Error
  Out Bus Element7 : Outport  PortName=ID51_DeltaQ  Element=MessageStatus.Remote
  Out Bus Element8 : Outport  PortName=ID51_DeltaQ  Element=MessageStatus.Length
  Out Bus Element9 : Outport  PortName=ID51_DeltaQ  Element=MessageStatus.Status
  wires:
  Packed_ID51_DeltaQ_In/1 -> DeltaQ/1
  DeltaQ/1 -> Out Bus Element/1  "ID51_DeltaQ.DeltaQ1"
  DeltaQ/2 -> Out Bus Element1/1  "ID51_DeltaQ.DeltaQ2"
  DeltaQ/3 -> Out Bus Element2/1  "ID51_DeltaQ.DeltaQ3"
  DeltaQ/4 -> Out Bus Element3/1  "ID51_DeltaQ.DeltaQ4"
  DeltaQ/5 -> Out Bus Element4/1  "ID51_DeltaQ.MessageStatus.ID"
  DeltaQ/6 -> Out Bus Element5/1  "ID51_DeltaQ.MessageStatus.Timestamp"
  DeltaQ/7 -> Out Bus Element6/1  "ID51_DeltaQ.MessageStatus.Error"
  DeltaQ/8 -> Out Bus Element7/1  "ID51_DeltaQ.MessageStatus.Remote"
  DeltaQ/9 -> Out Bus Element8/1  "ID51_DeltaQ.MessageStatus.Length"
  DeltaQ/10 -> Out Bus Element9/1  "ID51_DeltaQ.MessageStatus.Status"

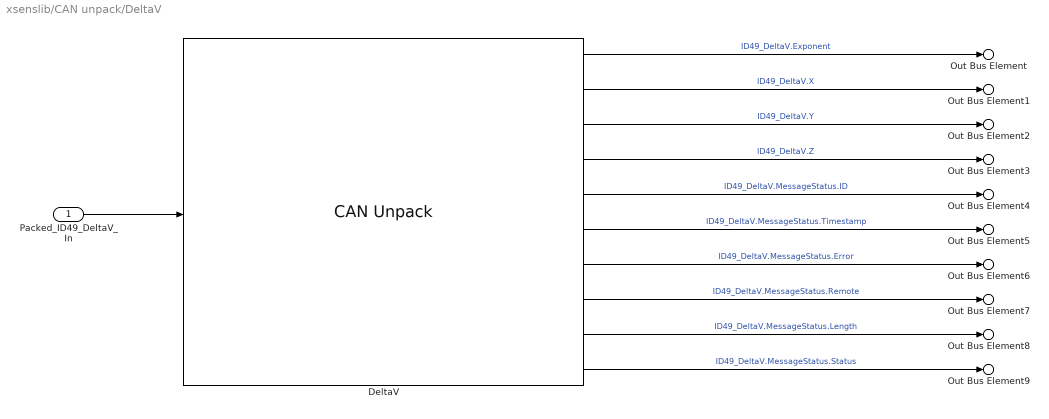
== system xsenslib/CAN unpack/DeltaV ==
  Packed_ID49_DeltaV_In : Inport
  DeltaV : canmsglib/CAN Unpack  CANdbFile=C:\Users\rodri\Dev\Projects\External\Tramontina\atlas\interface_models\xsens.dbc  MsgList=DeltaV  MsgName=DeltaV  MsgIDType=Standard (11-bit identifier)  MsgIdentifier=49  MsgLength=7  SignalInfo={'Exponent','48','8','BE','unsigned','Standard','0','1','0','-Inf','Inf';'X','8','16','BE','signed','Standard','0','7.6294e-06','0','-0.25','0.25';'Y','24','16','BE','signed','Standard','0','7.6294e-06','0','-0.25','0.25';'Z','40','16','BE','signed','Standard','0','7.6294e-06','0','-0.25','0.25'}  IDPort=on  TimestampPort=on  ErrorPort=on  RemotePort=on  LengthPort=on  StatusPort=on  ApplyMinMax=off
      settings: SourceProductBaseCode=XP,ME,VN
  Out Bus Element : Outport  PortName=ID49_DeltaV  Element=Exponent
  Out Bus Element1 : Outport  PortName=ID49_DeltaV  Element=X
  Out Bus Element2 : Outport  PortName=ID49_DeltaV  Element=Y
  Out Bus Element3 : Outport  PortName=ID49_DeltaV  Element=Z
  Out Bus Element4 : Outport  PortName=ID49_DeltaV  Element=MessageStatus.ID
  Out Bus Element5 : Outport  PortName=ID49_DeltaV  Element=MessageStatus.Timestamp
  Out Bus Element6 : Outport  PortName=ID49_DeltaV  Element=MessageStatus.Error
  Out Bus Element7 : Outport  PortName=ID49_DeltaV  Element=MessageStatus.Remote
  Out Bus Element8 : Outport  PortName=ID49_DeltaV  Element=MessageStatus.Length
  Out Bus Element9 : Outport  PortName=ID49_DeltaV  Element=MessageStatus.Status
  wires:
  Packed_ID49_DeltaV_In/1 -> DeltaV/1
  DeltaV/1 -> Out Bus Element/1  "ID49_DeltaV.Exponent"
  DeltaV/2 -> Out Bus Element1/1  "ID49_DeltaV.X"
  DeltaV/3 -> Out Bus Element2/1  "ID49_DeltaV.Y"
  DeltaV/4 -> Out Bus Element3/1  "ID49_DeltaV.Z"
  DeltaV/5 -> Out Bus Element4/1  "ID49_DeltaV.MessageStatus.ID"
  DeltaV/6 -> Out Bus Element5/1  "ID49_DeltaV.MessageStatus.Timestamp"
  DeltaV/7 -> Out Bus Element6/1  "ID49_DeltaV.MessageStatus.Error"
  DeltaV/8 -> Out Bus Element7/1  "ID49_DeltaV.MessageStatus.Remote"
  DeltaV/9 -> Out Bus Element8/1  "ID49_DeltaV.MessageStatus.Length"
  DeltaV/10 -> Out Bus Element9/1  "ID49_DeltaV.MessageStatus.Status"

== system xsenslib/CAN unpack/Error ==
  Packed_ID1_Error_In : Inport
  Error : canmsglib/CAN Unpack  CANdbFile=C:\Users\rodri\Dev\Projects\External\Tramontina\atlas\interface_models\xsens.dbc  MsgList=Error  MsgName=Error  MsgIDType=Standard (11-bit identifier)  MsgIdentifier=1  MsgLength=1  SignalInfo={}  IDPort=on  TimestampPort=on  ErrorPort=on  RemotePort=on  LengthPort=on  StatusPort=on  ApplyMinMax=off
      settings: SourceProductBaseCode=XP,ME,VN
  Out Bus Element : Outport  PortName=ID1_Error  Element=MessageStatus.ID
  Out Bus Element1 : Outport  PortName=ID1_Error  Element=MessageStatus.Timestamp
  Out Bus Element2 : Outport  PortName=ID1_Error  Element=MessageStatus.Error
  Out Bus Element3 : Outport  PortName=ID1_Error  Element=MessageStatus.Remote
  Out Bus Element4 : Outport  PortName=ID1_Error  Element=MessageStatus.Length
  Out Bus Element5 : Outport  PortName=ID1_Error  Element=MessageStatus.Status
  wires:
  Packed_ID1_Error_In/1 -> Error/1
  Error/1 -> Out Bus Element/1  "ID1_Error.MessageStatus.ID"
  Error/2 -> Out Bus Element1/1  "ID1_Error.MessageStatus.Timestamp"
  Error/3 -> Out Bus Element2/1  "ID1_Error.MessageStatus.Error"
  Error/4 -> Out Bus Element3/1  "ID1_Error.MessageStatus.Remote"
  Error/5 -> Out Bus Element4/1  "ID1_Error.MessageStatus.Length"
  Error/6 -> Out Bus Element5/1  "ID1_Error.MessageStatus.Status"

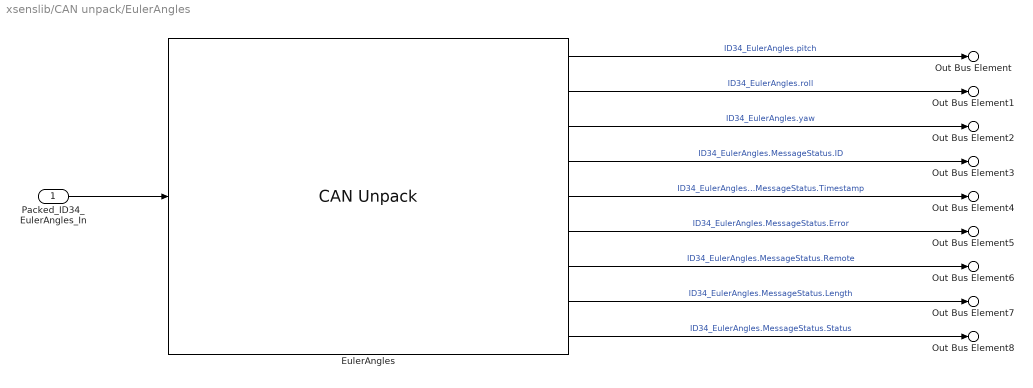
== system xsenslib/CAN unpack/EulerAngles ==
  Packed_ID34_EulerAngles_In : Inport
  EulerAngles : canmsglib/CAN Unpack  CANdbFile=C:\Users\rodri\Dev\Projects\External\Tramontina\atlas\interface_models\xsens.dbc  MsgList=EulerAngles  MsgName=EulerAngles  MsgIDType=Standard (11-bit identifier)  MsgIdentifier=34  MsgLength=6  SignalInfo={'pitch','24','16','BE','signed','Standard','0','0.0078125','0','-90','90';'roll','8','16','BE','signed','Standard','0','0.0078125','0','-180','180';'yaw','40','16','BE','signed','Standard','0','0.0078125','0','-180','180'}  IDPort=on  TimestampPort=on  ErrorPort=on  RemotePort=on  LengthPort=on  StatusPort=on  ApplyMinMax=off
      settings: SourceProductBaseCode=XP,ME,VN
  Out Bus Element : Outport  PortName=ID34_EulerAngles  Element=pitch
  Out Bus Element1 : Outport  PortName=ID34_EulerAngles  Element=roll
  Out Bus Element2 : Outport  PortName=ID34_EulerAngles  Element=yaw
  Out Bus Element3 : Outport  PortName=ID34_EulerAngles  Element=MessageStatus.ID
  Out Bus Element4 : Outport  PortName=ID34_EulerAngles  Element=MessageStatus.Timestamp
  Out Bus Element5 : Outport  PortName=ID34_EulerAngles  Element=MessageStatus.Error
  Out Bus Element6 : Outport  PortName=ID34_EulerAngles  Element=MessageStatus.Remote
  Out Bus Element7 : Outport  PortName=ID34_EulerAngles  Element=MessageStatus.Length
  Out Bus Element8 : Outport  PortName=ID34_EulerAngles  Element=MessageStatus.Status
  wires:
  Packed_ID34_EulerAngles_In/1 -> EulerAngles/1
  EulerAngles/1 -> Out Bus Element/1  "ID34_EulerAngles.pitch"
  EulerAngles/2 -> Out Bus Element1/1  "ID34_EulerAngles.roll"
  EulerAngles/3 -> Out Bus Element2/1  "ID34_EulerAngles.yaw"
  EulerAngles/4 -> Out Bus Element3/1  "ID34_EulerAngles.MessageStatus.ID"
  EulerAngles/5 -> Out Bus Element4/1  "ID34_EulerAngles.MessageStatus.Timestamp"
  EulerAngles/6 -> Out Bus Element5/1  "ID34_EulerAngles.MessageStatus.Error"
  EulerAngles/7 -> Out Bus Element6/1  "ID34_EulerAngles.MessageStatus.Remote"
  EulerAngles/8 -> Out Bus Element7/1  "ID34_EulerAngles.MessageStatus.Length"
  EulerAngles/9 -> Out Bus Element8/1  "ID34_EulerAngles.MessageStatus.Status"

== system xsenslib/CAN unpack/FreeAcceleration ==
  Packed_ID53_FreeAcceleration_In : Inport
  FreeAcceleration : canmsglib/CAN Unpack  CANdbFile=C:\Users\rodri\Dev\Projects\External\Tramontina\atlas\interface_models\xsens.dbc  MsgList=FreeAcceleration  MsgName=FreeAcceleration  MsgIDType=Standard (11-bit identifier)  MsgIdentifier=53  MsgLength=6  SignalInfo={'FreeAccX','8','16','BE','signed','Standard','0','0.0039062','0','-100','100';'FreeAccY','24','16','BE','signed','Standard','0','0.0039062','0','-100','100';'FreeAccZ','40','16','BE','signed','Standard','0','0.0039062','0','-100','100'}  IDPort=on  TimestampPort=on  ErrorPort=on  RemotePort=on  LengthPort=on  StatusPort=on  ApplyMinMax=off
      settings: SourceProductBaseCode=XP,ME,VN
  Out Bus Element : Outport  PortName=ID53_FreeAcceleration  Element=FreeAccX
  Out Bus Element1 : Outport  PortName=ID53_FreeAcceleration  Element=FreeAccY
  Out Bus Element2 : Outport  PortName=ID53_FreeAcceleration  Element=FreeAccZ
  Out Bus Element3 : Outport  PortName=ID53_FreeAcceleration  Element=MessageStatus.ID
  Out Bus Element4 : Outport  PortName=ID53_FreeAcceleration  Element=MessageStatus.Timestamp
  Out Bus Element5 : Outport  PortName=ID53_FreeAcceleration  Element=MessageStatus.Error
  Out Bus Element6 : Outport  PortName=ID53_FreeAcceleration  Element=MessageStatus.Remote
  Out Bus Element7 : Outport  PortName=ID53_FreeAcceleration  Element=MessageStatus.Length
  Out Bus Element8 : Outport  PortName=ID53_FreeAcceleration  Element=MessageStatus.Status
  wires:
  Packed_ID53_FreeAcceleration_In/1 -> FreeAcceleration/1
  FreeAcceleration/1 -> Out Bus Element/1  "ID53_FreeAcceleration.FreeAccX"
  FreeAcceleration/2 -> Out Bus Element1/1  "ID53_FreeAcceleration.FreeAccY"
  FreeAcceleration/3 -> Out Bus Element2/1  "ID53_FreeAcceleration.FreeAccZ"
  FreeAcceleration/4 -> Out Bus Element3/1  "ID53_FreeAcceleration.MessageStatus.ID"
  FreeAcceleration/5 -> Out Bus Element4/1  "ID53_FreeAcceleration.MessageStatus.Timestamp"
  FreeAcceleration/6 -> Out Bus Element5/1  "ID53_FreeAcceleration.MessageStatus.Error"
  FreeAcceleration/7 -> Out Bus Element6/1  "ID53_FreeAcceleration.MessageStatus.Remote"
  FreeAcceleration/8 -> Out Bus Element7/1  "ID53_FreeAcceleration.MessageStatus.Length"
  FreeAcceleration/9 -> Out Bus Element8/1  "ID53_FreeAcceleration.MessageStatus.Status"

== system xsenslib/CAN unpack/GroupCounter ==
  Packed_ID6_GroupCounter_In : Inport
  GroupCounter : canmsglib/CAN Unpack  CANdbFile=C:\Users\rodri\Dev\Projects\External\Tramontina\atlas\interface_models\xsens.dbc  MsgList=GroupCounter  MsgName=GroupCounter  MsgIDType=Standard (11-bit identifier)  MsgIdentifier=6  MsgLength=2  SignalInfo={'Counter','8','16','BE','unsigned','Standard','0','1','0','-Inf','Inf'}  IDPort=on  TimestampPort=on  ErrorPort=on  RemotePort=on  LengthPort=on  StatusPort=on  ApplyMinMax=off
      settings: SourceProductBaseCode=XP,ME,VN
  Out Bus Element : Outport  PortName=ID6_GroupCounter  Element=Counter
  Out Bus Element1 : Outport  PortName=ID6_GroupCounter  Element=MessageStatus.ID
  Out Bus Element2 : Outport  PortName=ID6_GroupCounter  Element=MessageStatus.Timestamp
  Out Bus Element3 : Outport  PortName=ID6_GroupCounter  Element=MessageStatus.Error
  Out Bus Element4 : Outport  PortName=ID6_GroupCounter  Element=MessageStatus.Remote
  Out Bus Element5 : Outport  PortName=ID6_GroupCounter  Element=MessageStatus.Length
  Out Bus Element6 : Outport  PortName=ID6_GroupCounter  Element=MessageStatus.Status
  wires:
  Packed_ID6_GroupCounter_In/1 -> GroupCounter/1
  GroupCounter/1 -> Out Bus Element/1  "ID6_GroupCounter.Counter"
  GroupCounter/2 -> Out Bus Element1/1  "ID6_GroupCounter.MessageStatus.ID"
  GroupCounter/3 -> Out Bus Element2/1  "ID6_GroupCounter.MessageStatus.Timestamp"
  GroupCounter/4 -> Out Bus Element3/1  "ID6_GroupCounter.MessageStatus.Error"
  GroupCounter/5 -> Out Bus Element4/1  "ID6_GroupCounter.MessageStatus.Remote"
  GroupCounter/6 -> Out Bus Element5/1  "ID6_GroupCounter.MessageStatus.Length"
  GroupCounter/7 -> Out Bus Element6/1  "ID6_GroupCounter.MessageStatus.Status"
